simulink model "CLAHEExample"  (R2019b)
settings: Solver=FixedStepDiscrete  StartTime=0.0  StopTime=402*324  FixedStep=1  RelTol=1e-3
PreLoadFcn:
  | % Initialize input image size
  | img = [240 320];
  | 
  | % Number of tiles fixed to 8 x 8
  | numTiles = [8 8];
  | 
  | % Initialize clip limit
  | normClipLimit  = 0.01;
  | 
  | % Number of Bins
  | numBins = 256;
  | 
  | dimI = [240 320] ;
  | 
  | dimTiles = dimI ./ numTiles;
  | 
  | numPixInTile = prod(dimTiles);
  | 
  | minClipLimit = ceil(numPixInTile/numBins);
  | 
  | clipLimit = minClipLimit + round(normClipLimit*(numPixInTile-minClipLimit));
  | 
  | % Initialize value for 1-D lookup table
  | tabVal = uint8(floor(numBins./(1:numBins-1)));
  | 
  | % Initialize wordlength and fractionlength
  | normFact1 = fi(1/(dimTiles(1)*dimTiles(2)/4),0);
  | 
  | normFact2 = fi(1/(prod(dimTiles)/2),0);
  | 
  | normFact3 = fi(1/(prod(dimTiles)),0);
  | 
  | grayxval = (numBins-1)/numPixInTile;
  | fi_grayxval = fi(grayxval,0);
InitFcn:
  | img = imread(get_param('CLAHEExample/inputImage','FileName'));
  | %img = [240 320];
  | numTiles = [8 8];
  | 
  | normClipLimit = str2double(get_param('CLAHEExample/CLAHEHDLAlgorithm','normClipLimit'));
  | 
  | numBins = 256;
  | 
  | dimI = size(img);
  | 
  | dimTiles = dimI ./ numTiles;
  | 
  | numPixInTile = prod(dimTiles);
  | 
  | minClipLimit = ceil(numPixInTile/numBins);
  | 
  | clipLimit = minClipLimit + round(normClipLimit*(numPixInTile-minClipLimit));
  | 
  | tabVal = uint8(floor(numBins./(1:numBins-1)));
  | 
  | normFact1 = fi(1/(dimTiles(1)*dimTiles(2)/4),0);
  | 
  | normFact2 = fi(1/(prod(dimTiles)/2),0);
  | 
  | normFact3 = fi(1/(prod(dimTiles)),0);
  | 
  | grayxval = (numBins-1)/numPixInTile;
  | fi_grayxval = fi(grayxval,0);
libraries: simulink x64, hdlsllib x46, visionhdlutilities x9, visionhdlstatistics x2, visionhdlio x2, visionsources x1
(part 3 of 3)

== system CLAHEExample/CLAHEHDLAlgorithm/histoEqPipeline/histPipe2/redistribute ==
  histoIn : Inport
  totalExcess : Inport  Port=2
  active : Inport  Port=3
  valid : Inport  Port=4
  1-D Lookup Table1 : Lookup_n-D  NumberOfTableDimensions=1  LookupTableObject=''  BreakpointsForDimension1=[1:255]  BreakpointsForDimension1FirstPoint=10  BreakpointsForDimension2FirstPoint=10  BreakpointsForDimension1Spacing=12  BreakpointsForDimension2Spacing=12  IndexSearchMethod=Evenly spaced points  Table=tabVal  InterpMethod=Flat  DiagnosticForOutOfRangeInput=Error  RemoveProtectionInput=on  InternalRulePriority=Speed  OutDataTypeStr=uint8  RndMeth=Simplest  SaturateOnIntegerOverflow=on  InputSameDT=on
  Add : Sum  OutDataTypeStr=fixdt(0,ceil(log2(numPixInTile)),0)
  Add1 : Sum  Inputs=-+
  Bus Creator : BusCreator  Inputs=5
  Compare To Constant1 : simulink/Logic and Bit Operations/Compare To Constant  relop=<  const=clipLimit  OutDataTypeStr=boolean
  Data Type Conversion : DataTypeConversion  OutDataTypeStr=uint8
  Delay{,1,3,5} (4 alike) : Delay  DelayLength=1
  Logical Operator3 : Logic  AllPortsSameDT=off  OutDataTypeStr=boolean
  Logical Operator4 : Logic  AllPortsSameDT=off  OutDataTypeStr=boolean
  MATLAB Function1 : MATLAB Function  TreatAsAtomicUnit=on
  Switch : Switch  Criteria=u2 ~= 0
  Switch1 : Switch  Criteria=u2 ~= 0
  excessFeedback : Switch  Criteria=u2 ~= 0
  ramBus : Outport  VectorParamsAs1DForOutWhenUnconnected=off
  done : Outport  Port=2  VectorParamsAs1DForOutWhenUnconnected=off
  wires:
  Add/1 -> Switch/1
  Add1/1 -> Switch1/1
  totalExcess/1 -> excessFeedback/3
  excessFeedback/1 -> MATLAB Function1/2(excessIn), Switch1/3, Add1/2
  Delay/1 -> excessFeedback/1
  Switch1/1 -> Delay/1
  histoIn/1 -> Add/1, Switch/3, Compare To Constant1/1
  Switch/1 -> Bus Creator/1  "histVal"
  Bus Creator/1 -> ramBus/1
  Delay3/1 -> Bus Creator/3  "wr_en"
  Delay5/1 -> Bus Creator/2  "wr_addr"
  MATLAB Function1/4(done) -> done/1
  MATLAB Function1/3(rdValid) -> Delay3/1, Bus Creator/5  "rd_valid"
  MATLAB Function1/2(rdAddr) -> Bus Creator/4, Delay5/1  "rd_addr"
  Compare To Constant1/1 -> Logical Operator3/1
  Logical Operator3/1 -> Switch/2, Switch1/2
  valid/1 -> Logical Operator4/1
  Logical Operator4/1 -> Logical Operator3/2
  active/1 -> MATLAB Function1/1(active), Logical Operator4/2, excessFeedback/2
  MATLAB Function1/1(binIncr) -> Add1/1, Add/2
  MATLAB Function1/5(excessOut) -> Data Type Conversion/1
  1-D Lookup Table1/1 -> Delay1/1
  Delay1/1 -> MATLAB Function1/3(stepIn)
  Data Type Conversion/1 -> 1-D Lookup Table1/1

== system CLAHEExample/CLAHEHDLAlgorithm/tileGeneration/histResetBuffer/pixelBusGenerator ==
  reset : Inport
  validIn : Inport  Port=2
  Horizontal : hdlsllib/Sources/HDL Counter  CountType=Count limited  CountInit=0  CountStep=1  CountMax=hEnd  CountFromType=Initial value  CountFrom=0  CountResetPort=on  CountLoadPort=off  CountEnbPort=on  CountDirPort=off  CountDataType=Unsigned  CountWordLen=ceil(log2(hEnd))  CountFracLen=0  CountSampTime=1
      settings: SourceProductName=Simulink
  Logical Operator{3..6} (4 alike) : Logic  AllPortsSameDT=off  OutDataTypeStr=boolean
  Pixel Control Bus Creator : visionhdlutilities/Pixel Control Bus Creator
      settings: SourceProductName=Vision HDL Toolbox  SourceProductBaseCode=VT
  Vertical : hdlsllib/Sources/HDL Counter  CountType=Count limited  CountInit=0  CountStep=1  CountMax=vEnd  CountFromType=Initial value  CountFrom=0  CountResetPort=on  CountLoadPort=off  CountEnbPort=on  CountDirPort=off  CountDataType=Unsigned  CountWordLen=ceil(log2(vEnd))  CountFracLen=0  CountSampTime=1
      settings: SourceProductName=Simulink
  hEnd : simulink/Logic and Bit Operations/Compare To Constant  relop===  const=hEnd  OutDataTypeStr=boolean
  hStart : simulink/Logic and Bit Operations/Compare To Constant  relop===  const=0  OutDataTypeStr=boolean
  vEnd : simulink/Logic and Bit Operations/Compare To Constant  relop===  const=vEnd  OutDataTypeStr=boolean
  vStart : simulink/Logic and Bit Operations/Compare To Constant  relop===  const=0  OutDataTypeStr=boolean
  busOut : Outport  VectorParamsAs1DForOutWhenUnconnected=off
  wires:
  validIn/1 -> Pixel Control Bus Creator/5, Logical Operator4/1, Logical Operator5/1, Logical Operator6/1, Logical Operator3/1, Horizontal/2, Vertical/2
  Horizontal/1 -> hEnd/1, hStart/1
  hEnd/1 -> Logical Operator4/2
  Vertical/1 -> vStart/1, vEnd/1
  vStart/1 -> Logical Operator5/2
  vEnd/1 -> Logical Operator6/2
  Logical Operator5/1 -> Pixel Control Bus Creator/3
  Logical Operator3/1 -> Pixel Control Bus Creator/1
  Logical Operator4/1 -> Pixel Control Bus Creator/2
  hStart/1 -> Logical Operator3/2
  Logical Operator6/1 -> Pixel Control Bus Creator/4
  Pixel Control Bus Creator/1 -> busOut/1
  reset/1 -> Vertical/1, Horizontal/1

== system CLAHEExample/CLAHEHDLAlgorithm/histoEqPipeline/histPipe1/histoExcess/Subsystem1 ==
  Constant : Constant  Value=0  OutDataTypeStr=boolean  SampleTime=-1
  Pixel Control Bus Creator : visionhdlutilities/Pixel Control Bus Creator
      settings: SourceProductName=Vision HDL Toolbox  SourceProductBaseCode=VT
  Out1 : Outport  VectorParamsAs1DForOutWhenUnconnected=off
  wires:
  Constant/1 -> Pixel Control Bus Creator/2, Pixel Control Bus Creator/3, Pixel Control Bus Creator/4, Pixel Control Bus Creator/5, Pixel Control Bus Creator/1
  Pixel Control Bus Creator/1 -> Out1/1

== system CLAHEExample/CLAHEHDLAlgorithm/histoEqPipeline/histPipe2/histoExcess/Subsystem1 ==
  Constant : Constant  Value=0  OutDataTypeStr=boolean  SampleTime=-1
  Pixel Control Bus Creator : visionhdlutilities/Pixel Control Bus Creator
      settings: SourceProductName=Vision HDL Toolbox  SourceProductBaseCode=VT
  Out1 : Outport  VectorParamsAs1DForOutWhenUnconnected=off
  wires:
  Constant/1 -> Pixel Control Bus Creator/2, Pixel Control Bus Creator/3, Pixel Control Bus Creator/4, Pixel Control Bus Creator/5, Pixel Control Bus Creator/1
  Pixel Control Bus Creator/1 -> Out1/1

== matlab function CLAHEExample/CLAHEHDLAlgorithm/histoEqPipeline/histPipe1/redistribute/MATLAB Function1 ==
  data: active input; binIncr output; excessIn input; stepIn input; rdAddr output; rdValid output; done output; excessOut output
function [binIncr, rdAddr, rdValid, done, excessOut] = redistributeCtrl(active, excessIn, stepIn)
%#codegen

% Create persistent variables
persistent state
persistent addr valid excess step k incr addr_overflow

% Initialize variables
if isempty(state)
    state = uint8(0);
    addr = uint16(0);
    valid = false;
    excess = uint16(0);
    step = uint8(0);
    k = uint8(0);
    incr = uint8(0);
    addr_overflow = uint16(0);
end

% Define states for Master State Machine
S1 = uint8(0); % IDLE/EXCESSIN
S2 = uint8(1); % STEPCALC
S3 = uint8(2); % RDADDR
S4 = uint8(3); % STOP
S5 = uint8(4); % 

switch (state)
    case S1
        binIncr = uint8(0);
        rdAddr = uint8(0);
        rdValid = false;
        done = false;
        excessOut = uint16(0);
        
        addr = uint16(0);
        valid = false;
        excess = uint16(excessIn);
        step = uint8(0);
        k = uint8(k);
        incr = uint8(0);
        addr_overflow = uint16(0);
        
        if (active)
            state = S2;
        else
            state = S1;
        end
        
    case S2
        if excess >= uint16(256)
            binIncr = uint8(bitsra(excess,8));
        else
            binIncr = uint8(1);
        end
        rdAddr = uint8(k);
        rdValid = valid;
        done = false;
        excessOut = uint16(excess);
        
        addr = uint16(k);
        valid = false;
        excess = uint16(excess);
        step = uint8(0);
        k = uint8(k);
        incr = uint8(binIncr);
        addr_overflow = uint16(0);
        
        state = S3;
    
    case S3
        binIncr = uint8(incr);
        rdAddr = uint8(k);
        rdValid = valid;
        done = false;
        excessOut = uint16(excess);
        
        addr = uint16(k);
        valid = true;
        excess = uint16(excess);
        step = uint8(stepIn);
        k = uint8(k);
        incr = uint8(incr);
        addr_overflow = uint16(0);
        
        state = S4;
        
    case S4
        binIncr = uint8(incr);
        rdAddr = uint8(addr);
        rdValid = valid;
        done = false;
        excessOut = uint16(excess);
        
        if addr_overflow > 255 || excessIn == uint16(0)
            if excessIn == uint16(0)
                state = S5;
            else
                state = S1;
            end
            addr = uint16(0);
            valid = false;
            k = uint8(k+1);
        else
            state = S4;
            addr = uint16(addr + uint16(step));
            valid = true;
            k = uint8(k);
        end
        
        incr = uint8(binIncr);
        excess = uint16(excess);
        step = uint8(stepIn);
        addr_overflow = uint16(addr + uint16(step));
        
    case S5
        binIncr = uint8(0);
        rdAddr = uint8(0);
        rdValid = false;
        done = true;
        excessOut = uint16(0);
        
        addr = uint16(0);
        valid = false;
        excess = uint16(0);
        step = uint8(0);
        k = uint8(0);
        incr = uint8(binIncr);
        
        state = S1;
       
    otherwise
        binIncr = uint8(0);
        rdAddr = uint8(0);
        rdValid = false;
        done = false;
        excessOut = uint16(0);
        
        addr = uint16(0);
        valid = false;
        excess = uint16(0);
        step = uint8(0);
        k = uint8(0);
        incr = uint8(0);
        
        state = S1;
end

== matlab function CLAHEExample/CLAHEHDLAlgorithm/histoEqPipeline/histPipe2/redistribute/MATLAB Function1 ==
  data: active input; binIncr output; excessIn input; stepIn input; rdAddr output; rdValid output; done output; excessOut output
function [binIncr, rdAddr, rdValid, done, excessOut] = redistributeCtrl(active, excessIn, stepIn)
%#codegen

% Create persistent variables
persistent state
persistent addr valid excess step k incr addr_overflow

% Initialize variables
if isempty(state)
    state = uint8(0);
    addr = uint16(0);
    valid = false;
    excess = uint16(0);
    step = uint8(0);
    k = uint8(0);
    incr = uint8(0);
    addr_overflow = uint16(0);
end

% Define states for Master State Machine
S1 = uint8(0); % IDLE/EXCESSIN
S2 = uint8(1); % STEPCALC
S3 = uint8(2); % RDADDR
S4 = uint8(3); % STOP
S5 = uint8(4); % 

switch (state)
    case S1
        binIncr = uint8(0);
        rdAddr = uint8(0);
        rdValid = false;
        done = false;
        excessOut = uint16(0);
        
        addr = uint16(0);
        valid = false;
        excess = uint16(excessIn);
        step = uint8(0);
        k = uint8(k);
        incr = uint8(0);
        addr_overflow = uint16(0);
        
        if (active)
            state = S2;
        else
            state = S1;
        end
        
    case S2
        if excess >= uint16(256)
            binIncr = uint8(bitsra(excess,8));
        else
            binIncr = uint8(1);
        end
        rdAddr = uint8(k);
        rdValid = valid;
        done = false;
        excessOut = uint16(excess);
        
        addr = uint16(k);
        valid = false;
        excess = uint16(excess);
        step = uint8(0);
        k = uint8(k);
        incr = uint8(binIncr);
        addr_overflow = uint16(0);
        
        state = S3;
    
    case S3
        binIncr = uint8(incr);
        rdAddr = uint8(k);
        rdValid = valid;
        done = false;
        excessOut = uint16(excess);
        
        addr = uint16(k);
        valid = true;
        excess = uint16(excess);
        step = uint8(stepIn);
        k = uint8(k);
        incr = uint8(incr);
        addr_overflow = uint16(0);
        
        state = S4;
        
    case S4
        binIncr = uint8(incr);
        rdAddr = uint8(addr);
        rdValid = valid;
        done = false;
        excessOut = uint16(excess);
        
        if addr_overflow > 255 || excessIn == uint16(0)
            if excessIn == uint16(0)
                state = S5;
            else
                state = S1;
            end
            addr = uint16(0);
            valid = false;
            k = uint8(k+1);
        else
            state = S4;
            addr = uint16(addr + uint16(step));
            valid = true;
            k = uint8(k);
        end
        
        incr = uint8(binIncr);
        excess = uint16(excess);
        step = uint8(stepIn);
        addr_overflow = uint16(addr + uint16(step));
        
    case S5
        binIncr = uint8(0);
        rdAddr = uint8(0);
        rdValid = false;
        done = true;
        excessOut = uint16(0);
        
        addr = uint16(0);
        valid = false;
        excess = uint16(0);
        step = uint8(0);
        k = uint8(0);
        incr = uint8(binIncr);
        
        state = S1;
       
    otherwise
        binIncr = uint8(0);
        rdAddr = uint8(0);
        rdValid = false;
        done = false;
        excessOut = uint16(0);
        
        addr = uint16(0);
        valid = false;
        excess = uint16(0);
        step = uint8(0);
        k = uint8(0);
        incr = uint8(0);
        
        state = S1;
end
